simulink model "mpc555rt_multitasking"  (Simulink 6.0)
settings: Solver=FixedStepDiscrete  SolverMode=MultiTasking  StartTime=0.0  StopTime=100  FixedStep=T_mpc555_multitasking  RelTol=1e-3
PreLoadFcn:
  | RTWConfigurationCB('preloadfcn', bdroot);
  | T_mpc555_multitasking = 0.001;
InitFcn:
  | % START RTW CONFIGURATION CODE %
  | RTWConfigurationCB('rtw_target_initfcn',gcs);
  | % END RTW CONFIGURATION CODE %
libraries: exprofilelib x8, mpc555drivers x2, canblocks x1, mpc555toucan x1
settings Model: Creator=The MathWorks Inc.  LastModifiedBy=batserve  ExtModeAutoUpdateStatusClock=off  BufferReuse=off  ProdHWDeviceType=Motorola PowerPC
settings DataIOCC: SignalLoggingName=sigsOut
settings OptimizationCC: InlineParams=on  InlineInvariantSignals=off  OptimizeBlockIOStorage=off  BufferReuse=off  EnforceIntegerDowncast=off  ExpressionFolding=off  FoldNonRolledExpr=off  LocalBlockOutputs=off  OptimizeModelRefInitCode=on  LifeSpan=1
settings DebuggingCC: CheckExecutionContextPreStartOutputMsg=on  CheckExecutionContextRuntimeOutputMsg=on  SolverPrmCheckMsg=none
settings HardwareCC: ProdEndianess=BigEndian  ProdHWDeviceType=Motorola PowerPC  TargetHWDeviceType=32-bit Generic
settings ModelReferenceCC: UpdateModelReferenceTargets=IfOutOfDate
settings RTWCC: SystemTargetFile=mpc555rt.tlc  TemplateMakefile=mpc555rt.tmf  Description=Embedded Target for Motorola MPC555 (real-time target)  ProcessScript=mpc555rt_make_rtw_hook
settings CodeAppCC: IgnoreCustomStorageClasses=off
settings STFCustomTargetCC: TargetFcnLib=ansi_tfl_tmw.mat  GenFloatMathFcnCalls=ANSI_C  ModelReferenceCompliant=off  CombineOutputUpdateFcns=on  ERTCustomFileBanners=on  SystemTargetFile=mpc555rt.tlc
settings ERTTargetCC: TargetFcnLib=ansi_tfl_tmw.mat  GenFloatMathFcnCalls=ANSI_C  ModelReferenceCompliant=off  SupportContinuousTime=on  SupportNonInlinedSFcns=on  RootIOFormat=Individual Arguments  ERTCustomFileTemplate=example_file_process.tlc  InitialValueSource=Model
settings CustomProperty: DataType=RTWOptions_EnumType__toolbox_rtw_targets_mpc555dk_mpc555dk_mpc555rt_MPC555_OPTIMIZATION_SWITCH  Value=speed
settings EnumStrPairs: String=speed

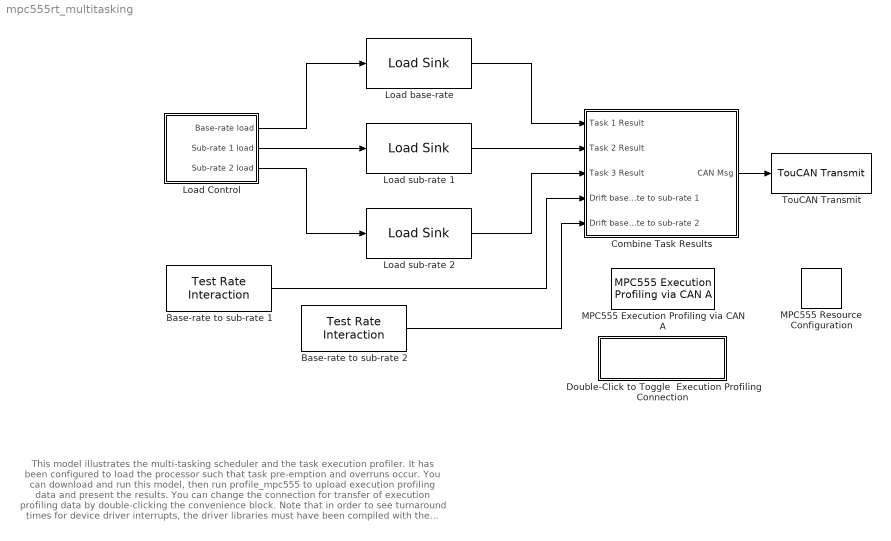
== system mpc555rt_multitasking ==
  note: This model illustrates the multi-tasking scheduler and the task execution profiler. It has
      | been configured to load the processor such that task pre-emption and overruns occur.
      |
      | You can download and run this model, then run profile_mpc555 to upload execution profiling
      | data  and present the results.  You can change the connection for transfer of execution
      | profiling data by double-clicking the convenience block.
      |
      | Note that in order to see turnaround times for device driver interrupts, the driver libraries must
      | have been compiled with the PROFILING_ENABLED flag set to 1.
  Base-rate to sub-rate 1 : exprofilelib/Test Rate Interaction  t=T_mpc555_multitasking
  Base-rate to sub-rate 2 : exprofilelib/Test Rate Interaction  t=T_mpc555_multitasking*4
  Combine Task Results : Subsystem  PropExecContextAcrossSSBoundary=on
  Double-Click to Toggle  Execution Profiling Connection : Subsystem  TreatAsAtomicUnit=on  PropExecContextAcrossSSBoundary=on
      settings: OpenFcn=toggle_exprofiling_mpc555(gcs);
      mask Display: disp('Execution Profiling\nis currently over CAN');
  Load Control : Subsystem  PropExecContextAcrossSSBoundary=on
  Load base-rate : exprofilelib/Load Sink  mode=single  t=T_mpc555_multitasking
  Load sub-rate 1 : exprofilelib/Load Sink  mode=single  t=T_mpc555_multitasking*4
  Load sub-rate 2 : exprofilelib/Load Sink  mode=single  t=T_mpc555_multitasking*16
  MPC555 Resource Configuration : mpc555drivers/MPC555 Resource Configuration  Tag=RTW CONFIGURATION BLOCK  Priority=-100000  oldParentName=mpc555rt_multitasking  oldBlockName=|  defaultConfigLibrary=mpc555drivers
      | mpc555rt_multitasking/MPC555
      | Resource
      | Configuration
  MPC555 Execution Profiling via CAN A : mpc555drivers/Execution Profiling/MPC555 Execution Profiling via CAN A  commandId=hex2dec('1FFFFF00')  execCopyFcn=on  dataId=hex2dec('1FFFFF01')  t=T_mpc555_multitasking*4
  TouCAN Transmit : mpc555toucan/TouCAN Transmit  module=A  tx_mode=Queued transmission with shared buffer  fifo_queue_length=8  bufferids=0  t=-1  enablePassThru=off
  wires:
  Load Control/1(Base-rate load) -> Load base-rate/1
  Load base-rate/1 -> Combine Task Results/1(Task 1 Result)
  Load Control/2(Sub-rate 1 load) -> Load sub-rate 1/1
  Load Control/3(Sub-rate 2 load) -> Load sub-rate 2/1
  Load sub-rate 1/1 -> Combine Task Results/2(Task 2 Result)
  Load sub-rate 2/1 -> Combine Task Results/3(Task 3 Result)
  Combine Task Results/1(CAN Msg) -> TouCAN Transmit/1
  Base-rate to sub-rate 1/1 -> Combine Task Results/4(Drift base-rate to sub-rate 1)
  Base-rate to sub-rate 2/1 -> Combine Task Results/5(Drift base-rate to sub-rate 2)

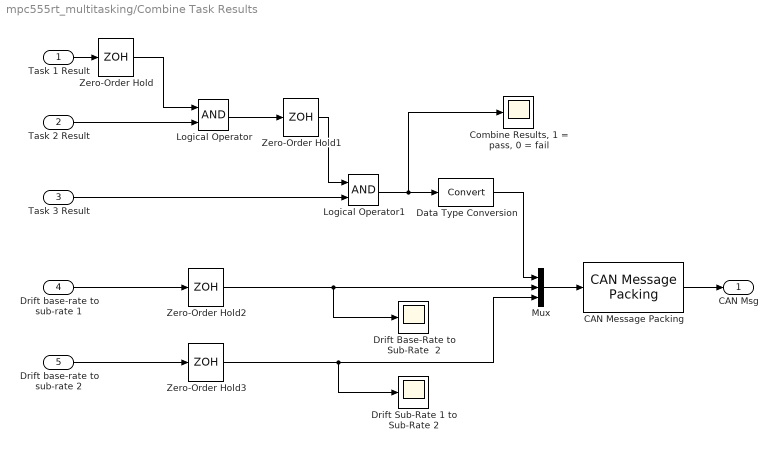
== system mpc555rt_multitasking/Combine Task Results ==
  Task 1 Result : Inport  Port=1  LatchInput=off
  Task 2 Result : Inport  Port=2  LatchInput=off
  Task 3 Result : Inport  Port=3  LatchInput=off
  Drift base-rate to sub-rate 1 : Inport  Port=4  LatchInput=off
  Drift base-rate to sub-rate 2 : Inport  Port=5  LatchInput=off
  CAN Message Packing : canblocks/CAN Message Packing  id=hex2dec('1')  message_type=Extended (29-bit identifier)  endian=Big Endian (Motorola)
  "Combine Results, 1 = pass, 0 = fail" : Scope
      settings: TimeRange=0.1  YMin=0.95  YMax=1.05  SaveName=ScopeData12
  Data Type Conversion : DataTypeConversion  OutDataTypeMode=uint8  RndMeth=Zero
  Drift Base-Rate to Sub-Rate  2 : Scope
      settings: TimeRange=20  YMin=-1  YMax=1
  Drift Sub-Rate 1 to Sub-Rate 2 : Scope
      settings: TimeRange=20  YMin=-1  YMax=1
  Logical Operator : Logic  AllPortsSameDT=off
  Logical Operator1 : Logic  AllPortsSameDT=off
  Mux : Mux  Inputs=3
  Zero-Order Hold : ZeroOrderHold  SampleTime=T_mpc555_multitasking*4
  Zero-Order Hold1 : ZeroOrderHold  SampleTime=T_mpc555_multitasking*16
  Zero-Order Hold2 : ZeroOrderHold  SampleTime=T_mpc555_multitasking*16
  Zero-Order Hold3 : ZeroOrderHold  SampleTime=T_mpc555_multitasking*16
  CAN Msg : Outport
  wires:
  Zero-Order Hold/1 -> Logical Operator/1
  Logical Operator/1 -> Zero-Order Hold1/1
  Logical Operator1/1 -> "Combine Results, 1 = pass, 0 = fail"/1, Data Type Conversion/1
  Zero-Order Hold1/1 -> Logical Operator1/1
  CAN Message Packing/1 -> CAN Msg/1
  Task 1 Result/1 -> Zero-Order Hold/1
  Task 2 Result/1 -> Logical Operator/2
  Task 3 Result/1 -> Logical Operator1/2
  Mux/1 -> CAN Message Packing/1
  Data Type Conversion/1 -> Mux/1
  Drift base-rate to sub-rate 1/1 -> Zero-Order Hold2/1
  Drift base-rate to sub-rate 2/1 -> Zero-Order Hold3/1
  Zero-Order Hold2/1 -> Drift Base-Rate to Sub-Rate  2/1, Mux/2
  Zero-Order Hold3/1 -> Mux/3, Drift Sub-Rate 1 to Sub-Rate 2/1

== system mpc555rt_multitasking/Double-Click to Toggle  Execution Profiling Connection ==

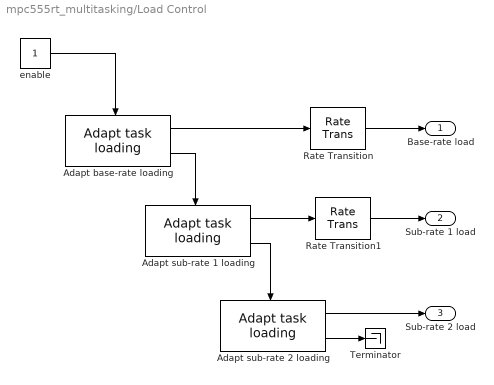
== system mpc555rt_multitasking/Load Control ==
  Adapt base-rate loading : exprofilelib/Adapt task loading  rateNum=0  target=uint32(1250)  adapt=2  t=T_mpc555_multitasking*16
  Adapt sub-rate 1 loading : exprofilelib/Adapt task loading  rateNum=1  target=uint32(5000)  adapt=8  t=T_mpc555_multitasking*16
  Adapt sub-rate 2 loading : exprofilelib/Adapt task loading  rateNum=2  target=uint32(20000)  adapt=32  t=T_mpc555_multitasking*16
  Rate Transition : RateTransition
  Rate Transition1 : RateTransition
  Terminator : Terminator
  enable : Constant  OutDataTypeMode=boolean
  Base-rate load : Outport
  Sub-rate 1 load : Outport  Port=2
  Sub-rate 2 load : Outport  Port=3
  wires:
  Rate Transition/1 -> Base-rate load/1
  Adapt base-rate loading/1 -> Rate Transition/1
  enable/1 -> Adapt base-rate loading/Enable
  Adapt base-rate loading/2 -> Adapt sub-rate 1 loading/Enable
  Rate Transition1/1 -> Sub-rate 1 load/1
  Adapt sub-rate 1 loading/1 -> Rate Transition1/1
  Adapt sub-rate 1 loading/2 -> Adapt sub-rate 2 loading/Enable
  Adapt sub-rate 2 loading/1 -> Sub-rate 2 load/1
  Adapt sub-rate 2 loading/2 -> Terminator/1
